simulink model "Campus_Power_System_updated"  (R2024a)
settings: Solver=daessc  StartTime=0.0  StopTime=1  RelTol=1e-3
libraries: spsThreePhaseVIMeasurementLib x57, spsThreePhaseTransformerTwoWindingsLib x56, spsThreePhaseSeriesRLCLoadLib x55, spsThreePhasePISectionLineLib x54, spsThreePhaseBreakerLib x9, spsCurrentMeasurementLib x3, spsMultimeterLib x1, spsThreePhaseSourceLib x1, spsThreePhaseFaultLib x1, sps_lib x1
(part 2 of 3)

== system Campus_Power_System_updated/Engineering (1) ==
  33/11KV Transformer 1 : spsThreePhaseTransformerTwoWindingsLib/Three-Phase Transformer (Two Windings)  Winding1Connection=Yg  Winding2Connection=Yg  CoreType=Three single-phase transformers  SetSaturation=off  Hysteresis=off  DataFile='hysteresis'  SetInitialFlux=off  Measurements=None  UNITS=pu  NominalPower=[ 250e6 , 50 ]  Winding1=[33e3 , 0.002 , 0.08 ]  Winding2=[ 11e3 , 0.002 , 0.08 ]  Rm=500  Lm=500  L0=0.5  Saturation=[ 0,0 ; 0.0024,1.2 ; 1.0,1.52 ]  InitialFluxes=[ 0.8 , -0.8 , 0.7 ]  BreakLoop=off  DiscreteSolver=Trapezoidal iterative  DataType=off  TransfoNumber=1
  BUS1 : spsThreePhaseVIMeasurementLib/Three-Phase V-I Measurement  VoltageMeasurement=phase-to-ground  SetLabelV=off  LabelV=Vabc  Vpu=off  VpuLL=off  CurrentMeasurement=yes  SetLabelI=off  LabelI=Iabc  Ipu=off  Pbase=100e6  Vbase=500e3  OutputType=Complex  PhasorSimulation=off  PSBequivalent=0
  Mux1 : Mux  Inputs=2
  Scope1 : Scope
  Three-Phase Series RLC Load : spsThreePhaseSeriesRLCLoadLib/Three-Phase Series RLC Load  LConnTagsString=A|B|C  Configuration=Y (grounded)  NominalVoltage=1000  Vabc=[1e3 1e3 1e3]  Vabcp=[1e3 1e3 1e3]  NominalFrequency=60  UnbalancedPower=off  ActivePower=10e3  InductivePower=100  CapacitivePower=100  Pabc=[10e3 9e3 11e3]  QLabc=[100 90 110]  QCabc=[100 90 110]  Pabcp=[10e3 9e3 11e3]  QLabcp=[100 90 110]  QCabcp=[100 90 110]  Measurements=None  LoadType=constant Z
  A : PMIOPort  Side=Left
  B : PMIOPort  Port=2  Side=Left
  C : PMIOPort  Port=3  Side=Left
  wires:
  BUS1/2 -> Mux1/2
  BUS1/1 -> Mux1/1
  Mux1/1 -> Scope1/1
  connections:
  33/11KV Transformer 1/RConn3 -- BUS1/LConn3
  33/11KV Transformer 1/RConn1 -- BUS1/LConn1
  BUS1/RConn2 -- Three-Phase Series RLC Load/LConn2
  BUS1/RConn3 -- Three-Phase Series RLC Load/LConn3
  33/11KV Transformer 1/RConn2 -- BUS1/LConn2
  BUS1/RConn1 -- Three-Phase Series RLC Load/LConn1
  33/11KV Transformer 1/LConn1 -- A/RConn1
  33/11KV Transformer 1/LConn3 -- C/RConn1
  33/11KV Transformer 1/LConn2 -- B/RConn1

== system Campus_Power_System_updated/Engineering (ii) ==
  33/11KV Transformer 1 : spsThreePhaseTransformerTwoWindingsLib/Three-Phase Transformer (Two Windings)  Winding1Connection=Yg  Winding2Connection=Yg  CoreType=Three single-phase transformers  SetSaturation=off  Hysteresis=off  DataFile='hysteresis'  SetInitialFlux=off  Measurements=None  UNITS=pu  NominalPower=[ 250e6 , 50 ]  Winding1=[33e3 , 0.002 , 0.08 ]  Winding2=[ 11e3 , 0.002 , 0.08 ]  Rm=500  Lm=500  L0=0.5  Saturation=[ 0,0 ; 0.0024,1.2 ; 1.0,1.52 ]  InitialFluxes=[ 0.8 , -0.8 , 0.7 ]  BreakLoop=off  DiscreteSolver=Trapezoidal iterative  DataType=off  TransfoNumber=1
  BUS1 : spsThreePhaseVIMeasurementLib/Three-Phase V-I Measurement  VoltageMeasurement=phase-to-ground  SetLabelV=off  LabelV=Vabc  Vpu=off  VpuLL=off  CurrentMeasurement=yes  SetLabelI=off  LabelI=Iabc  Ipu=off  Pbase=100e6  Vbase=500e3  OutputType=Complex  PhasorSimulation=off  PSBequivalent=0
  Mux1 : Mux  Inputs=2
  Scope1 : Scope
  Three-Phase Series RLC Load : spsThreePhaseSeriesRLCLoadLib/Three-Phase Series RLC Load  LConnTagsString=A|B|C  Configuration=Y (grounded)  NominalVoltage=1000  Vabc=[1e3 1e3 1e3]  Vabcp=[1e3 1e3 1e3]  NominalFrequency=60  UnbalancedPower=off  ActivePower=10e3  InductivePower=100  CapacitivePower=100  Pabc=[10e3 9e3 11e3]  QLabc=[100 90 110]  QCabc=[100 90 110]  Pabcp=[10e3 9e3 11e3]  QLabcp=[100 90 110]  QCabcp=[100 90 110]  Measurements=None  LoadType=constant Z
  A : PMIOPort  Side=Left
  B : PMIOPort  Port=2  Side=Left
  C : PMIOPort  Port=3  Side=Left
  wires:
  BUS1/2 -> Mux1/2
  BUS1/1 -> Mux1/1
  Mux1/1 -> Scope1/1
  connections:
  33/11KV Transformer 1/RConn3 -- BUS1/LConn3
  33/11KV Transformer 1/RConn1 -- BUS1/LConn1
  BUS1/RConn2 -- Three-Phase Series RLC Load/LConn2
  BUS1/RConn3 -- Three-Phase Series RLC Load/LConn3
  33/11KV Transformer 1/RConn2 -- BUS1/LConn2
  BUS1/RConn1 -- Three-Phase Series RLC Load/LConn1
  33/11KV Transformer 1/LConn1 -- A/RConn1
  33/11KV Transformer 1/LConn3 -- C/RConn1
  33/11KV Transformer 1/LConn2 -- B/RConn1

== system Campus_Power_System_updated/Environmental Science ==
  33/11KV Transformer 1 : spsThreePhaseTransformerTwoWindingsLib/Three-Phase Transformer (Two Windings)  Winding1Connection=Yg  Winding2Connection=Yg  CoreType=Three single-phase transformers  SetSaturation=off  Hysteresis=off  DataFile='hysteresis'  SetInitialFlux=off  Measurements=None  UNITS=pu  NominalPower=[ 250e6 , 50 ]  Winding1=[33e3 , 0.002 , 0.08 ]  Winding2=[ 11e3 , 0.002 , 0.08 ]  Rm=500  Lm=500  L0=0.5  Saturation=[ 0,0 ; 0.0024,1.2 ; 1.0,1.52 ]  InitialFluxes=[ 0.8 , -0.8 , 0.7 ]  BreakLoop=off  DiscreteSolver=Trapezoidal iterative  DataType=off  TransfoNumber=1
  Environmental Science : Scope
  Environmental Science_ : spsThreePhaseVIMeasurementLib/Three-Phase V-I Measurement  VoltageMeasurement=phase-to-ground  SetLabelV=off  LabelV=Vabc  Vpu=off  VpuLL=off  CurrentMeasurement=yes  SetLabelI=off  LabelI=Iabc  Ipu=off  Pbase=100e6  Vbase=500e3  OutputType=Complex  PhasorSimulation=off  PSBequivalent=0
  Mux1 : Mux  Inputs=2
  Three-Phase Series RLC Load : spsThreePhaseSeriesRLCLoadLib/Three-Phase Series RLC Load  LConnTagsString=A|B|C  Configuration=Y (grounded)  NominalVoltage=240  Vabc=[1e3 1e3 1e3]  Vabcp=[1e3 1e3 1e3]  NominalFrequency=50  UnbalancedPower=off  ActivePower=10e3  InductivePower=100  CapacitivePower=100  Pabc=[10e3 9e3 11e3]  QLabc=[100 90 110]  QCabc=[100 90 110]  Pabcp=[10e3 9e3 11e3]  QLabcp=[100 90 110]  QCabcp=[100 90 110]  Measurements=None  LoadType=constant Z
  A : PMIOPort  Side=Left
  B : PMIOPort  Port=2  Side=Left
  C : PMIOPort  Port=3  Side=Left
  wires:
  Environmental Science_/2 -> Mux1/2
  Environmental Science_/1 -> Mux1/1
  Mux1/1 -> Environmental Science/1
  connections:
  33/11KV Transformer 1/RConn3 -- Environmental Science_/LConn3
  33/11KV Transformer 1/RConn1 -- Environmental Science_/LConn1
  Environmental Science_/RConn2 -- Three-Phase Series RLC Load/LConn2
  Environmental Science_/RConn3 -- Three-Phase Series RLC Load/LConn3
  33/11KV Transformer 1/RConn2 -- Environmental Science_/LConn2
  Environmental Science_/RConn1 -- Three-Phase Series RLC Load/LConn1
  33/11KV Transformer 1/LConn1 -- A/RConn1
  33/11KV Transformer 1/LConn3 -- C/RConn1
  33/11KV Transformer 1/LConn2 -- B/RConn1

== system Campus_Power_System_updated/Guest House ==
  33/11KV Transformer 1 : spsThreePhaseTransformerTwoWindingsLib/Three-Phase Transformer (Two Windings)  Winding1Connection=Yg  Winding2Connection=Yg  CoreType=Three single-phase transformers  SetSaturation=off  Hysteresis=off  DataFile='hysteresis'  SetInitialFlux=off  Measurements=None  UNITS=pu  NominalPower=[ 250e6 , 50 ]  Winding1=[33e3 , 0.002 , 0.08 ]  Winding2=[ 11e3 , 0.002 , 0.08 ]  Rm=500  Lm=500  L0=0.5  Saturation=[ 0,0 ; 0.0024,1.2 ; 1.0,1.52 ]  InitialFluxes=[ 0.8 , -0.8 , 0.7 ]  BreakLoop=off  DiscreteSolver=Trapezoidal iterative  DataType=off  TransfoNumber=1
  BUS1 : spsThreePhaseVIMeasurementLib/Three-Phase V-I Measurement  VoltageMeasurement=phase-to-ground  SetLabelV=off  LabelV=Vabc  Vpu=off  VpuLL=off  CurrentMeasurement=yes  SetLabelI=off  LabelI=Iabc  Ipu=off  Pbase=100e6  Vbase=500e3  OutputType=Complex  PhasorSimulation=off  PSBequivalent=0
  Mux1 : Mux  Inputs=2
  Scope1 : Scope
  Three-Phase Series RLC Load : spsThreePhaseSeriesRLCLoadLib/Three-Phase Series RLC Load  LConnTagsString=A|B|C  Configuration=Y (grounded)  NominalVoltage=1000  Vabc=[1e3 1e3 1e3]  Vabcp=[1e3 1e3 1e3]  NominalFrequency=60  UnbalancedPower=off  ActivePower=10e3  InductivePower=100  CapacitivePower=100  Pabc=[10e3 9e3 11e3]  QLabc=[100 90 110]  QCabc=[100 90 110]  Pabcp=[10e3 9e3 11e3]  QLabcp=[100 90 110]  QCabcp=[100 90 110]  Measurements=None  LoadType=constant Z
  A : PMIOPort  Side=Left
  B : PMIOPort  Port=2  Side=Left
  C : PMIOPort  Port=3  Side=Left
  wires:
  BUS1/2 -> Mux1/2
  BUS1/1 -> Mux1/1
  Mux1/1 -> Scope1/1
  connections:
  33/11KV Transformer 1/RConn3 -- BUS1/LConn3
  33/11KV Transformer 1/RConn1 -- BUS1/LConn1
  BUS1/RConn2 -- Three-Phase Series RLC Load/LConn2
  BUS1/RConn3 -- Three-Phase Series RLC Load/LConn3
  33/11KV Transformer 1/RConn2 -- BUS1/LConn2
  BUS1/RConn1 -- Three-Phase Series RLC Load/LConn1
  33/11KV Transformer 1/LConn1 -- A/RConn1
  33/11KV Transformer 1/LConn3 -- C/RConn1
  33/11KV Transformer 1/LConn2 -- B/RConn1

== system Campus_Power_System_updated/HRDB ==
  33/11KV Transformer 1 : spsThreePhaseTransformerTwoWindingsLib/Three-Phase Transformer (Two Windings)  Winding1Connection=Yg  Winding2Connection=Yg  CoreType=Three single-phase transformers  SetSaturation=off  Hysteresis=off  DataFile='hysteresis'  SetInitialFlux=off  Measurements=None  UNITS=pu  NominalPower=[ 250e6 , 50 ]  Winding1=[33e3 , 0.002 , 0.08 ]  Winding2=[ 11e3 , 0.002 , 0.08 ]  Rm=500  Lm=500  L0=0.5  Saturation=[ 0,0 ; 0.0024,1.2 ; 1.0,1.52 ]  InitialFluxes=[ 0.8 , -0.8 , 0.7 ]  BreakLoop=off  DiscreteSolver=Trapezoidal iterative  DataType=off  TransfoNumber=1
  BUS1 : spsThreePhaseVIMeasurementLib/Three-Phase V-I Measurement  VoltageMeasurement=phase-to-ground  SetLabelV=off  LabelV=Vabc  Vpu=off  VpuLL=off  CurrentMeasurement=yes  SetLabelI=off  LabelI=Iabc  Ipu=off  Pbase=100e6  Vbase=500e3  OutputType=Complex  PhasorSimulation=off  PSBequivalent=0
  Mux1 : Mux  Inputs=2
  Scope1 : Scope
  Three-Phase Series RLC Load : spsThreePhaseSeriesRLCLoadLib/Three-Phase Series RLC Load  LConnTagsString=A|B|C  Configuration=Y (grounded)  NominalVoltage=1000  Vabc=[1e3 1e3 1e3]  Vabcp=[1e3 1e3 1e3]  NominalFrequency=60  UnbalancedPower=off  ActivePower=10e3  InductivePower=100  CapacitivePower=100  Pabc=[10e3 9e3 11e3]  QLabc=[100 90 110]  QCabc=[100 90 110]  Pabcp=[10e3 9e3 11e3]  QLabcp=[100 90 110]  QCabcp=[100 90 110]  Measurements=None  LoadType=constant Z
  A : PMIOPort  Side=Left
  B : PMIOPort  Port=2  Side=Left
  C : PMIOPort  Port=3  Side=Left
  wires:
  BUS1/2 -> Mux1/2
  BUS1/1 -> Mux1/1
  Mux1/1 -> Scope1/1
  connections:
  33/11KV Transformer 1/RConn3 -- BUS1/LConn3
  33/11KV Transformer 1/RConn1 -- BUS1/LConn1
  BUS1/RConn2 -- Three-Phase Series RLC Load/LConn2
  BUS1/RConn3 -- Three-Phase Series RLC Load/LConn3
  33/11KV Transformer 1/RConn2 -- BUS1/LConn2
  BUS1/RConn1 -- Three-Phase Series RLC Load/LConn1
  33/11KV Transformer 1/LConn1 -- A/RConn1
  33/11KV Transformer 1/LConn3 -- C/RConn1
  33/11KV Transformer 1/LConn2 -- B/RConn1

== system Campus_Power_System_updated/HV laboratory ==
  33/11KV Transformer 1 : spsThreePhaseTransformerTwoWindingsLib/Three-Phase Transformer (Two Windings)  Winding1Connection=Yg  Winding2Connection=Yg  CoreType=Three single-phase transformers  SetSaturation=off  Hysteresis=off  DataFile='hysteresis'  SetInitialFlux=off  Measurements=None  UNITS=pu  NominalPower=[ 250e6 , 50 ]  Winding1=[33e3 , 0.002 , 0.08 ]  Winding2=[ 11e3 , 0.002 , 0.08 ]  Rm=500  Lm=500  L0=0.5  Saturation=[ 0,0 ; 0.0024,1.2 ; 1.0,1.52 ]  InitialFluxes=[ 0.8 , -0.8 , 0.7 ]  BreakLoop=off  DiscreteSolver=Trapezoidal iterative  DataType=off  TransfoNumber=1
  BUS1 : spsThreePhaseVIMeasurementLib/Three-Phase V-I Measurement  VoltageMeasurement=phase-to-ground  SetLabelV=off  LabelV=Vabc  Vpu=off  VpuLL=off  CurrentMeasurement=yes  SetLabelI=off  LabelI=Iabc  Ipu=off  Pbase=100e6  Vbase=500e3  OutputType=Complex  PhasorSimulation=off  PSBequivalent=0
  Mux1 : Mux  Inputs=2
  Scope1 : Scope
  Three-Phase Series RLC Load : spsThreePhaseSeriesRLCLoadLib/Three-Phase Series RLC Load  LConnTagsString=A|B|C  Configuration=Y (grounded)  NominalVoltage=1000  Vabc=[1e3 1e3 1e3]  Vabcp=[1e3 1e3 1e3]  NominalFrequency=60  UnbalancedPower=off  ActivePower=10e3  InductivePower=100  CapacitivePower=100  Pabc=[10e3 9e3 11e3]  QLabc=[100 90 110]  QCabc=[100 90 110]  Pabcp=[10e3 9e3 11e3]  QLabcp=[100 90 110]  QCabcp=[100 90 110]  Measurements=None  LoadType=constant Z
  A : PMIOPort  Side=Left
  B : PMIOPort  Port=2  Side=Left
  C : PMIOPort  Port=3  Side=Left
  wires:
  BUS1/2 -> Mux1/2
  BUS1/1 -> Mux1/1
  Mux1/1 -> Scope1/1
  connections:
  33/11KV Transformer 1/RConn3 -- BUS1/LConn3
  33/11KV Transformer 1/RConn1 -- BUS1/LConn1
  BUS1/RConn2 -- Three-Phase Series RLC Load/LConn2
  BUS1/RConn3 -- Three-Phase Series RLC Load/LConn3
  33/11KV Transformer 1/RConn2 -- BUS1/LConn2
  BUS1/RConn1 -- Three-Phase Series RLC Load/LConn1
  33/11KV Transformer 1/LConn1 -- A/RConn1
  33/11KV Transformer 1/LConn3 -- C/RConn1
  33/11KV Transformer 1/LConn2 -- B/RConn1

== system Campus_Power_System_updated/Health Centre ==
  33/11KV Transformer 1 : spsThreePhaseTransformerTwoWindingsLib/Three-Phase Transformer (Two Windings)  Winding1Connection=Yg  Winding2Connection=Yg  CoreType=Three single-phase transformers  SetSaturation=off  Hysteresis=off  DataFile='hysteresis'  SetInitialFlux=off  Measurements=None  UNITS=pu  NominalPower=[ 250e6 , 50 ]  Winding1=[33e3 , 0.002 , 0.08 ]  Winding2=[ 11e3 , 0.002 , 0.08 ]  Rm=500  Lm=500  L0=0.5  Saturation=[ 0,0 ; 0.0024,1.2 ; 1.0,1.52 ]  InitialFluxes=[ 0.8 , -0.8 , 0.7 ]  BreakLoop=off  DiscreteSolver=Trapezoidal iterative  DataType=off  TransfoNumber=1
  BUS1 : spsThreePhaseVIMeasurementLib/Three-Phase V-I Measurement  VoltageMeasurement=phase-to-ground  SetLabelV=off  LabelV=Vabc  Vpu=off  VpuLL=off  CurrentMeasurement=yes  SetLabelI=off  LabelI=Iabc  Ipu=off  Pbase=100e6  Vbase=500e3  OutputType=Complex  PhasorSimulation=off  PSBequivalent=0
  Mux1 : Mux  Inputs=2
  Scope1 : Scope
  Three-Phase Series RLC Load : spsThreePhaseSeriesRLCLoadLib/Three-Phase Series RLC Load  LConnTagsString=A|B|C  Configuration=Y (grounded)  NominalVoltage=1000  Vabc=[1e3 1e3 1e3]  Vabcp=[1e3 1e3 1e3]  NominalFrequency=60  UnbalancedPower=off  ActivePower=10e3  InductivePower=100  CapacitivePower=100  Pabc=[10e3 9e3 11e3]  QLabc=[100 90 110]  QCabc=[100 90 110]  Pabcp=[10e3 9e3 11e3]  QLabcp=[100 90 110]  QCabcp=[100 90 110]  Measurements=None  LoadType=constant Z
  A : PMIOPort  Side=Left
  B : PMIOPort  Port=2  Side=Left
  C : PMIOPort  Port=3  Side=Left
  wires:
  BUS1/2 -> Mux1/2
  BUS1/1 -> Mux1/1
  Mux1/1 -> Scope1/1
  connections:
  33/11KV Transformer 1/RConn3 -- BUS1/LConn3
  33/11KV Transformer 1/RConn1 -- BUS1/LConn1
  BUS1/RConn2 -- Three-Phase Series RLC Load/LConn2
  BUS1/RConn3 -- Three-Phase Series RLC Load/LConn3
  33/11KV Transformer 1/RConn2 -- BUS1/LConn2
  BUS1/RConn1 -- Three-Phase Series RLC Load/LConn1
  33/11KV Transformer 1/LConn1 -- A/RConn1
  33/11KV Transformer 1/LConn3 -- C/RConn1
  33/11KV Transformer 1/LConn2 -- B/RConn1

== system Campus_Power_System_updated/Henry cafe ==
  33/11KV Transformer 1 : spsThreePhaseTransformerTwoWindingsLib/Three-Phase Transformer (Two Windings)  Winding1Connection=Yg  Winding2Connection=Yg  CoreType=Three single-phase transformers  SetSaturation=off  Hysteresis=off  DataFile='hysteresis'  SetInitialFlux=off  Measurements=None  UNITS=pu  NominalPower=[ 250e6 , 50 ]  Winding1=[33e3 , 0.002 , 0.08 ]  Winding2=[ 11e3 , 0.002 , 0.08 ]  Rm=500  Lm=500  L0=0.5  Saturation=[ 0,0 ; 0.0024,1.2 ; 1.0,1.52 ]  InitialFluxes=[ 0.8 , -0.8 , 0.7 ]  BreakLoop=off  DiscreteSolver=Trapezoidal iterative  DataType=off  TransfoNumber=1
  BUS1 : spsThreePhaseVIMeasurementLib/Three-Phase V-I Measurement  VoltageMeasurement=phase-to-ground  SetLabelV=off  LabelV=Vabc  Vpu=off  VpuLL=off  CurrentMeasurement=yes  SetLabelI=off  LabelI=Iabc  Ipu=off  Pbase=100e6  Vbase=500e3  OutputType=Complex  PhasorSimulation=off  PSBequivalent=0
  Mux1 : Mux  Inputs=2
  Scope1 : Scope
  Three-Phase Series RLC Load : spsThreePhaseSeriesRLCLoadLib/Three-Phase Series RLC Load  LConnTagsString=A|B|C  Configuration=Y (grounded)  NominalVoltage=1000  Vabc=[1e3 1e3 1e3]  Vabcp=[1e3 1e3 1e3]  NominalFrequency=60  UnbalancedPower=off  ActivePower=10e3  InductivePower=100  CapacitivePower=100  Pabc=[10e3 9e3 11e3]  QLabc=[100 90 110]  QCabc=[100 90 110]  Pabcp=[10e3 9e3 11e3]  QLabcp=[100 90 110]  QCabcp=[100 90 110]  Measurements=None  LoadType=constant Z
  A : PMIOPort  Side=Left
  B : PMIOPort  Port=2  Side=Left
  C : PMIOPort  Port=3  Side=Left
  wires:
  BUS1/2 -> Mux1/2
  BUS1/1 -> Mux1/1
  Mux1/1 -> Scope1/1
  connections:
  33/11KV Transformer 1/RConn3 -- BUS1/LConn3
  33/11KV Transformer 1/RConn1 -- BUS1/LConn1
  BUS1/RConn2 -- Three-Phase Series RLC Load/LConn2
  BUS1/RConn3 -- Three-Phase Series RLC Load/LConn3
  33/11KV Transformer 1/RConn2 -- BUS1/LConn2
  BUS1/RConn1 -- Three-Phase Series RLC Load/LConn1
  33/11KV Transformer 1/LConn1 -- A/RConn1
  33/11KV Transformer 1/LConn3 -- C/RConn1
  33/11KV Transformer 1/LConn2 -- B/RConn1

== system Campus_Power_System_updated/High Rise Block (Auxilliary) ==
  33/11KV Transformer 1 : spsThreePhaseTransformerTwoWindingsLib/Three-Phase Transformer (Two Windings)  Winding1Connection=Yg  Winding2Connection=Yg  CoreType=Three single-phase transformers  SetSaturation=off  Hysteresis=off  DataFile='hysteresis'  SetInitialFlux=off  Measurements=None  UNITS=pu  NominalPower=[ 250e6 , 50 ]  Winding1=[33e3 , 0.002 , 0.08 ]  Winding2=[ 11e3 , 0.002 , 0.08 ]  Rm=500  Lm=500  L0=0.5  Saturation=[ 0,0 ; 0.0024,1.2 ; 1.0,1.52 ]  InitialFluxes=[ 0.8 , -0.8 , 0.7 ]  BreakLoop=off  DiscreteSolver=Trapezoidal iterative  DataType=off  TransfoNumber=1
  BUS1 : spsThreePhaseVIMeasurementLib/Three-Phase V-I Measurement  VoltageMeasurement=phase-to-ground  SetLabelV=off  LabelV=Vabc  Vpu=off  VpuLL=off  CurrentMeasurement=yes  SetLabelI=off  LabelI=Iabc  Ipu=off  Pbase=100e6  Vbase=500e3  OutputType=Complex  PhasorSimulation=off  PSBequivalent=0
  Mux1 : Mux  Inputs=2
  Scope1 : Scope
  Three-Phase Series RLC Load : spsThreePhaseSeriesRLCLoadLib/Three-Phase Series RLC Load  LConnTagsString=A|B|C  Configuration=Y (grounded)  NominalVoltage=1000  Vabc=[1e3 1e3 1e3]  Vabcp=[1e3 1e3 1e3]  NominalFrequency=60  UnbalancedPower=off  ActivePower=10e3  InductivePower=100  CapacitivePower=100  Pabc=[10e3 9e3 11e3]  QLabc=[100 90 110]  QCabc=[100 90 110]  Pabcp=[10e3 9e3 11e3]  QLabcp=[100 90 110]  QCabcp=[100 90 110]  Measurements=None  LoadType=constant Z
  A : PMIOPort  Side=Left
  B : PMIOPort  Port=2  Side=Left
  C : PMIOPort  Port=3  Side=Left
  wires:
  BUS1/2 -> Mux1/2
  BUS1/1 -> Mux1/1
  Mux1/1 -> Scope1/1
  connections:
  33/11KV Transformer 1/RConn3 -- BUS1/LConn3
  33/11KV Transformer 1/RConn1 -- BUS1/LConn1
  BUS1/RConn2 -- Three-Phase Series RLC Load/LConn2
  BUS1/RConn3 -- Three-Phase Series RLC Load/LConn3
  33/11KV Transformer 1/RConn2 -- BUS1/LConn2
  BUS1/RConn1 -- Three-Phase Series RLC Load/LConn1
  33/11KV Transformer 1/LConn1 -- A/RConn1
  33/11KV Transformer 1/LConn3 -- C/RConn1
  33/11KV Transformer 1/LConn2 -- B/RConn1

== system Campus_Power_System_updated/High Rise Block A ==
  33/11KV Transformer 1 : spsThreePhaseTransformerTwoWindingsLib/Three-Phase Transformer (Two Windings)  Winding1Connection=Yg  Winding2Connection=Yg  CoreType=Three single-phase transformers  SetSaturation=off  Hysteresis=off  DataFile='hysteresis'  SetInitialFlux=off  Measurements=None  UNITS=pu  NominalPower=[ 250e6 , 50 ]  Winding1=[33e3 , 0.002 , 0.08 ]  Winding2=[ 11e3 , 0.002 , 0.08 ]  Rm=500  Lm=500  L0=0.5  Saturation=[ 0,0 ; 0.0024,1.2 ; 1.0,1.52 ]  InitialFluxes=[ 0.8 , -0.8 , 0.7 ]  BreakLoop=off  DiscreteSolver=Trapezoidal iterative  DataType=off  TransfoNumber=1
  BUS1 : spsThreePhaseVIMeasurementLib/Three-Phase V-I Measurement  VoltageMeasurement=phase-to-ground  SetLabelV=off  LabelV=Vabc  Vpu=off  VpuLL=off  CurrentMeasurement=yes  SetLabelI=off  LabelI=Iabc  Ipu=off  Pbase=100e6  Vbase=500e3  OutputType=Complex  PhasorSimulation=off  PSBequivalent=0
  Mux1 : Mux  Inputs=2
  Scope1 : Scope
  Three-Phase Series RLC Load : spsThreePhaseSeriesRLCLoadLib/Three-Phase Series RLC Load  LConnTagsString=A|B|C  Configuration=Y (grounded)  NominalVoltage=1000  Vabc=[1e3 1e3 1e3]  Vabcp=[1e3 1e3 1e3]  NominalFrequency=60  UnbalancedPower=off  ActivePower=10e3  InductivePower=100  CapacitivePower=100  Pabc=[10e3 9e3 11e3]  QLabc=[100 90 110]  QCabc=[100 90 110]  Pabcp=[10e3 9e3 11e3]  QLabcp=[100 90 110]  QCabcp=[100 90 110]  Measurements=None  LoadType=constant Z
  A : PMIOPort  Side=Left
  B : PMIOPort  Port=2  Side=Left
  C : PMIOPort  Port=3  Side=Left
  wires:
  BUS1/2 -> Mux1/2
  BUS1/1 -> Mux1/1
  Mux1/1 -> Scope1/1
  connections:
  33/11KV Transformer 1/RConn3 -- BUS1/LConn3
  33/11KV Transformer 1/RConn1 -- BUS1/LConn1
  BUS1/RConn2 -- Three-Phase Series RLC Load/LConn2
  BUS1/RConn3 -- Three-Phase Series RLC Load/LConn3
  33/11KV Transformer 1/RConn2 -- BUS1/LConn2
  BUS1/RConn1 -- Three-Phase Series RLC Load/LConn1
  33/11KV Transformer 1/LConn1 -- A/RConn1
  33/11KV Transformer 1/LConn3 -- C/RConn1
  33/11KV Transformer 1/LConn2 -- B/RConn1

== system Campus_Power_System_updated/High Rise Block B ==
  33/11KV Transformer 1 : spsThreePhaseTransformerTwoWindingsLib/Three-Phase Transformer (Two Windings)  Winding1Connection=Yg  Winding2Connection=Yg  CoreType=Three single-phase transformers  SetSaturation=off  Hysteresis=off  DataFile='hysteresis'  SetInitialFlux=off  Measurements=None  UNITS=pu  NominalPower=[ 250e6 , 50 ]  Winding1=[33e3 , 0.002 , 0.08 ]  Winding2=[ 11e3 , 0.002 , 0.08 ]  Rm=500  Lm=500  L0=0.5  Saturation=[ 0,0 ; 0.0024,1.2 ; 1.0,1.52 ]  InitialFluxes=[ 0.8 , -0.8 , 0.7 ]  BreakLoop=off  DiscreteSolver=Trapezoidal iterative  DataType=off  TransfoNumber=1
  BUS1 : spsThreePhaseVIMeasurementLib/Three-Phase V-I Measurement  VoltageMeasurement=phase-to-ground  SetLabelV=off  LabelV=Vabc  Vpu=off  VpuLL=off  CurrentMeasurement=yes  SetLabelI=off  LabelI=Iabc  Ipu=off  Pbase=100e6  Vbase=500e3  OutputType=Complex  PhasorSimulation=off  PSBequivalent=0
  Mux1 : Mux  Inputs=2
  Scope1 : Scope
  Three-Phase Series RLC Load : spsThreePhaseSeriesRLCLoadLib/Three-Phase Series RLC Load  LConnTagsString=A|B|C  Configuration=Y (grounded)  NominalVoltage=1000  Vabc=[1e3 1e3 1e3]  Vabcp=[1e3 1e3 1e3]  NominalFrequency=60  UnbalancedPower=off  ActivePower=10e3  InductivePower=100  CapacitivePower=100  Pabc=[10e3 9e3 11e3]  QLabc=[100 90 110]  QCabc=[100 90 110]  Pabcp=[10e3 9e3 11e3]  QLabcp=[100 90 110]  QCabcp=[100 90 110]  Measurements=None  LoadType=constant Z
  A : PMIOPort  Side=Left
  B : PMIOPort  Port=2  Side=Left
  C : PMIOPort  Port=3  Side=Left
  wires:
  BUS1/2 -> Mux1/2
  BUS1/1 -> Mux1/1
  Mux1/1 -> Scope1/1
  connections:
  33/11KV Transformer 1/RConn3 -- BUS1/LConn3
  33/11KV Transformer 1/RConn1 -- BUS1/LConn1
  BUS1/RConn2 -- Three-Phase Series RLC Load/LConn2
  BUS1/RConn3 -- Three-Phase Series RLC Load/LConn3
  33/11KV Transformer 1/RConn2 -- BUS1/LConn2
  BUS1/RConn1 -- Three-Phase Series RLC Load/LConn1
  33/11KV Transformer 1/LConn1 -- A/RConn1
  33/11KV Transformer 1/LConn3 -- C/RConn1
  33/11KV Transformer 1/LConn2 -- B/RConn1

== system Campus_Power_System_updated/High Rise Block C ==
  33/11KV Transformer 1 : spsThreePhaseTransformerTwoWindingsLib/Three-Phase Transformer (Two Windings)  Winding1Connection=Yg  Winding2Connection=Yg  CoreType=Three single-phase transformers  SetSaturation=off  Hysteresis=off  DataFile='hysteresis'  SetInitialFlux=off  Measurements=None  UNITS=pu  NominalPower=[ 250e6 , 50 ]  Winding1=[33e3 , 0.002 , 0.08 ]  Winding2=[ 11e3 , 0.002 , 0.08 ]  Rm=500  Lm=500  L0=0.5  Saturation=[ 0,0 ; 0.0024,1.2 ; 1.0,1.52 ]  InitialFluxes=[ 0.8 , -0.8 , 0.7 ]  BreakLoop=off  DiscreteSolver=Trapezoidal iterative  DataType=off  TransfoNumber=1
  BUS1 : spsThreePhaseVIMeasurementLib/Three-Phase V-I Measurement  VoltageMeasurement=phase-to-ground  SetLabelV=off  LabelV=Vabc  Vpu=off  VpuLL=off  CurrentMeasurement=yes  SetLabelI=off  LabelI=Iabc  Ipu=off  Pbase=100e6  Vbase=500e3  OutputType=Complex  PhasorSimulation=off  PSBequivalent=0
  Mux1 : Mux  Inputs=2
  Scope1 : Scope
  Three-Phase Series RLC Load : spsThreePhaseSeriesRLCLoadLib/Three-Phase Series RLC Load  LConnTagsString=A|B|C  Configuration=Y (grounded)  NominalVoltage=1000  Vabc=[1e3 1e3 1e3]  Vabcp=[1e3 1e3 1e3]  NominalFrequency=60  UnbalancedPower=off  ActivePower=10e3  InductivePower=100  CapacitivePower=100  Pabc=[10e3 9e3 11e3]  QLabc=[100 90 110]  QCabc=[100 90 110]  Pabcp=[10e3 9e3 11e3]  QLabcp=[100 90 110]  QCabcp=[100 90 110]  Measurements=None  LoadType=constant Z
  A : PMIOPort  Side=Left
  B : PMIOPort  Port=2  Side=Left
  C : PMIOPort  Port=3  Side=Left
  wires:
  BUS1/2 -> Mux1/2
  BUS1/1 -> Mux1/1
  Mux1/1 -> Scope1/1
  connections:
  33/11KV Transformer 1/RConn3 -- BUS1/LConn3
  33/11KV Transformer 1/RConn1 -- BUS1/LConn1
  BUS1/RConn2 -- Three-Phase Series RLC Load/LConn2
  BUS1/RConn3 -- Three-Phase Series RLC Load/LConn3
  33/11KV Transformer 1/RConn2 -- BUS1/LConn2
  BUS1/RConn1 -- Three-Phase Series RLC Load/LConn1
  33/11KV Transformer 1/LConn1 -- A/RConn1
  33/11KV Transformer 1/LConn3 -- C/RConn1
  33/11KV Transformer 1/LConn2 -- B/RConn1

== system Campus_Power_System_updated/Hydraulic Research Centre ==
  33/11KV Transformer 1 : spsThreePhaseTransformerTwoWindingsLib/Three-Phase Transformer (Two Windings)  Winding1Connection=Yg  Winding2Connection=Yg  CoreType=Three single-phase transformers  SetSaturation=off  Hysteresis=off  DataFile='hysteresis'  SetInitialFlux=off  Measurements=None  UNITS=pu  NominalPower=[ 250e6 , 50 ]  Winding1=[33e3 , 0.002 , 0.08 ]  Winding2=[ 11e3 , 0.002 , 0.08 ]  Rm=500  Lm=500  L0=0.5  Saturation=[ 0,0 ; 0.0024,1.2 ; 1.0,1.52 ]  InitialFluxes=[ 0.8 , -0.8 , 0.7 ]  BreakLoop=off  DiscreteSolver=Trapezoidal iterative  DataType=off  TransfoNumber=1
  BUS1 : spsThreePhaseVIMeasurementLib/Three-Phase V-I Measurement  VoltageMeasurement=phase-to-ground  SetLabelV=off  LabelV=Vabc  Vpu=off  VpuLL=off  CurrentMeasurement=yes  SetLabelI=off  LabelI=Iabc  Ipu=off  Pbase=100e6  Vbase=500e3  OutputType=Complex  PhasorSimulation=off  PSBequivalent=0
  Mux1 : Mux  Inputs=2
  Scope1 : Scope
  Three-Phase Series RLC Load : spsThreePhaseSeriesRLCLoadLib/Three-Phase Series RLC Load  LConnTagsString=A|B|C  Configuration=Y (grounded)  NominalVoltage=1000  Vabc=[1e3 1e3 1e3]  Vabcp=[1e3 1e3 1e3]  NominalFrequency=60  UnbalancedPower=off  ActivePower=10e3  InductivePower=100  CapacitivePower=100  Pabc=[10e3 9e3 11e3]  QLabc=[100 90 110]  QCabc=[100 90 110]  Pabcp=[10e3 9e3 11e3]  QLabcp=[100 90 110]  QCabcp=[100 90 110]  Measurements=None  LoadType=constant Z
  A : PMIOPort  Side=Left
  B : PMIOPort  Port=2  Side=Left
  C : PMIOPort  Port=3  Side=Left
  wires:
  BUS1/2 -> Mux1/2
  BUS1/1 -> Mux1/1
  Mux1/1 -> Scope1/1
  connections:
  33/11KV Transformer 1/RConn3 -- BUS1/LConn3
  33/11KV Transformer 1/RConn1 -- BUS1/LConn1
  BUS1/RConn2 -- Three-Phase Series RLC Load/LConn2
  BUS1/RConn3 -- Three-Phase Series RLC Load/LConn3
  33/11KV Transformer 1/RConn2 -- BUS1/LConn2
  BUS1/RConn1 -- Three-Phase Series RLC Load/LConn1
  33/11KV Transformer 1/LConn1 -- A/RConn1
  33/11KV Transformer 1/LConn3 -- C/RConn1
  33/11KV Transformer 1/LConn2 -- B/RConn1

== system Campus_Power_System_updated/Intercontinental Bank ==
  33/11KV Transformer 1 : spsThreePhaseTransformerTwoWindingsLib/Three-Phase Transformer (Two Windings)  Winding1Connection=Yg  Winding2Connection=Yg  CoreType=Three single-phase transformers  SetSaturation=off  Hysteresis=off  DataFile='hysteresis'  SetInitialFlux=off  Measurements=None  UNITS=pu  NominalPower=[ 250e6 , 50 ]  Winding1=[33e3 , 0.002 , 0.08 ]  Winding2=[ 11e3 , 0.002 , 0.08 ]  Rm=500  Lm=500  L0=0.5  Saturation=[ 0,0 ; 0.0024,1.2 ; 1.0,1.52 ]  InitialFluxes=[ 0.8 , -0.8 , 0.7 ]  BreakLoop=off  DiscreteSolver=Trapezoidal iterative  DataType=off  TransfoNumber=1
  BUS1 : spsThreePhaseVIMeasurementLib/Three-Phase V-I Measurement  VoltageMeasurement=phase-to-ground  SetLabelV=off  LabelV=Vabc  Vpu=off  VpuLL=off  CurrentMeasurement=yes  SetLabelI=off  LabelI=Iabc  Ipu=off  Pbase=100e6  Vbase=500e3  OutputType=Complex  PhasorSimulation=off  PSBequivalent=0
  Mux1 : Mux  Inputs=2
  Scope1 : Scope
  Three-Phase Series RLC Load : spsThreePhaseSeriesRLCLoadLib/Three-Phase Series RLC Load  LConnTagsString=A|B|C  Configuration=Y (grounded)  NominalVoltage=1000  Vabc=[1e3 1e3 1e3]  Vabcp=[1e3 1e3 1e3]  NominalFrequency=60  UnbalancedPower=off  ActivePower=10e3  InductivePower=100  CapacitivePower=100  Pabc=[10e3 9e3 11e3]  QLabc=[100 90 110]  QCabc=[100 90 110]  Pabcp=[10e3 9e3 11e3]  QLabcp=[100 90 110]  QCabcp=[100 90 110]  Measurements=None  LoadType=constant Z
  A : PMIOPort  Side=Left
  B : PMIOPort  Port=2  Side=Left
  C : PMIOPort  Port=3  Side=Left
  wires:
  BUS1/2 -> Mux1/2
  BUS1/1 -> Mux1/1
  Mux1/1 -> Scope1/1
  connections:
  33/11KV Transformer 1/RConn3 -- BUS1/LConn3
  33/11KV Transformer 1/RConn1 -- BUS1/LConn1
  BUS1/RConn2 -- Three-Phase Series RLC Load/LConn2
  BUS1/RConn3 -- Three-Phase Series RLC Load/LConn3
  33/11KV Transformer 1/RConn2 -- BUS1/LConn2
  BUS1/RConn1 -- Three-Phase Series RLC Load/LConn1
  33/11KV Transformer 1/LConn1 -- A/RConn1
  33/11KV Transformer 1/LConn3 -- C/RConn1
  33/11KV Transformer 1/LConn2 -- B/RConn1

== system Campus_Power_System_updated/International School ==
  33/11KV Transformer 1 : spsThreePhaseTransformerTwoWindingsLib/Three-Phase Transformer (Two Windings)  Winding1Connection=Yg  Winding2Connection=Yg  CoreType=Three single-phase transformers  SetSaturation=off  Hysteresis=off  DataFile='hysteresis'  SetInitialFlux=off  Measurements=None  UNITS=pu  NominalPower=[ 250e6 , 50 ]  Winding1=[33e3 , 0.002 , 0.08 ]  Winding2=[ 11e3 , 0.002 , 0.08 ]  Rm=500  Lm=500  L0=0.5  Saturation=[ 0,0 ; 0.0024,1.2 ; 1.0,1.52 ]  InitialFluxes=[ 0.8 , -0.8 , 0.7 ]  BreakLoop=off  DiscreteSolver=Trapezoidal iterative  DataType=off  TransfoNumber=1
  BUS1 : spsThreePhaseVIMeasurementLib/Three-Phase V-I Measurement  VoltageMeasurement=phase-to-ground  SetLabelV=off  LabelV=Vabc  Vpu=off  VpuLL=off  CurrentMeasurement=yes  SetLabelI=off  LabelI=Iabc  Ipu=off  Pbase=100e6  Vbase=500e3  OutputType=Complex  PhasorSimulation=off  PSBequivalent=0
  Mux1 : Mux  Inputs=2
  Scope1 : Scope
  Three-Phase Series RLC Load : spsThreePhaseSeriesRLCLoadLib/Three-Phase Series RLC Load  LConnTagsString=A|B|C  Configuration=Y (grounded)  NominalVoltage=1000  Vabc=[1e3 1e3 1e3]  Vabcp=[1e3 1e3 1e3]  NominalFrequency=60  UnbalancedPower=off  ActivePower=10e3  InductivePower=100  CapacitivePower=100  Pabc=[10e3 9e3 11e3]  QLabc=[100 90 110]  QCabc=[100 90 110]  Pabcp=[10e3 9e3 11e3]  QLabcp=[100 90 110]  QCabcp=[100 90 110]  Measurements=None  LoadType=constant Z
  A : PMIOPort  Side=Left
  B : PMIOPort  Port=2  Side=Left
  C : PMIOPort  Port=3  Side=Left
  wires:
  BUS1/2 -> Mux1/2
  BUS1/1 -> Mux1/1
  Mux1/1 -> Scope1/1
  connections:
  33/11KV Transformer 1/RConn3 -- BUS1/LConn3
  33/11KV Transformer 1/RConn1 -- BUS1/LConn1
  BUS1/RConn2 -- Three-Phase Series RLC Load/LConn2
  BUS1/RConn3 -- Three-Phase Series RLC Load/LConn3
  33/11KV Transformer 1/RConn2 -- BUS1/LConn2
  BUS1/RConn1 -- Three-Phase Series RLC Load/LConn1
  33/11KV Transformer 1/LConn1 -- A/RConn1
  33/11KV Transformer 1/LConn3 -- C/RConn1
  33/11KV Transformer 1/LConn2 -- B/RConn1

== system Campus_Power_System_updated/Jaja Hall ==
  33/11KV Transformer 1 : spsThreePhaseTransformerTwoWindingsLib/Three-Phase Transformer (Two Windings)  Winding1Connection=Yg  Winding2Connection=Yg  CoreType=Three single-phase transformers  SetSaturation=off  Hysteresis=off  DataFile='hysteresis'  SetInitialFlux=off  Measurements=None  UNITS=pu  NominalPower=[ 250e6 , 50 ]  Winding1=[33e3 , 0.002 , 0.08 ]  Winding2=[ 11e3 , 0.002 , 0.08 ]  Rm=500  Lm=500  L0=0.5  Saturation=[ 0,0 ; 0.0024,1.2 ; 1.0,1.52 ]  InitialFluxes=[ 0.8 , -0.8 , 0.7 ]  BreakLoop=off  DiscreteSolver=Trapezoidal iterative  DataType=off  TransfoNumber=1
  BUS1 : spsThreePhaseVIMeasurementLib/Three-Phase V-I Measurement  VoltageMeasurement=phase-to-ground  SetLabelV=off  LabelV=Vabc  Vpu=off  VpuLL=off  CurrentMeasurement=yes  SetLabelI=off  LabelI=Iabc  Ipu=off  Pbase=100e6  Vbase=500e3  OutputType=Complex  PhasorSimulation=off  PSBequivalent=0
  Mux1 : Mux  Inputs=2
  Scope1 : Scope
  Three-Phase Series RLC Load : spsThreePhaseSeriesRLCLoadLib/Three-Phase Series RLC Load  LConnTagsString=A|B|C  Configuration=Y (grounded)  NominalVoltage=1000  Vabc=[1e3 1e3 1e3]  Vabcp=[1e3 1e3 1e3]  NominalFrequency=60  UnbalancedPower=off  ActivePower=10e3  InductivePower=100  CapacitivePower=100  Pabc=[10e3 9e3 11e3]  QLabc=[100 90 110]  QCabc=[100 90 110]  Pabcp=[10e3 9e3 11e3]  QLabcp=[100 90 110]  QCabcp=[100 90 110]  Measurements=None  LoadType=constant Z
  A : PMIOPort  Side=Left
  B : PMIOPort  Port=2  Side=Left
  C : PMIOPort  Port=3  Side=Left
  wires:
  BUS1/2 -> Mux1/2
  BUS1/1 -> Mux1/1
  Mux1/1 -> Scope1/1
  connections:
  33/11KV Transformer 1/RConn3 -- BUS1/LConn3
  33/11KV Transformer 1/RConn1 -- BUS1/LConn1
  BUS1/RConn2 -- Three-Phase Series RLC Load/LConn2
  BUS1/RConn3 -- Three-Phase Series RLC Load/LConn3
  33/11KV Transformer 1/RConn2 -- BUS1/LConn2
  BUS1/RConn1 -- Three-Phase Series RLC Load/LConn1
  33/11KV Transformer 1/LConn1 -- A/RConn1
  33/11KV Transformer 1/LConn3 -- C/RConn1
  33/11KV Transformer 1/LConn2 -- B/RConn1

== system Campus_Power_System_updated/Kosoko Drive ==
  33/11KV Transformer 1 : spsThreePhaseTransformerTwoWindingsLib/Three-Phase Transformer (Two Windings)  Winding1Connection=Yg  Winding2Connection=Yg  CoreType=Three single-phase transformers  SetSaturation=off  Hysteresis=off  DataFile='hysteresis'  SetInitialFlux=off  Measurements=None  UNITS=pu  NominalPower=[ 250e6 , 50 ]  Winding1=[33e3 , 0.002 , 0.08 ]  Winding2=[ 11e3 , 0.002 , 0.08 ]  Rm=500  Lm=500  L0=0.5  Saturation=[ 0,0 ; 0.0024,1.2 ; 1.0,1.52 ]  InitialFluxes=[ 0.8 , -0.8 , 0.7 ]  BreakLoop=off  DiscreteSolver=Trapezoidal iterative  DataType=off  TransfoNumber=1
  BUS1 : spsThreePhaseVIMeasurementLib/Three-Phase V-I Measurement  VoltageMeasurement=phase-to-ground  SetLabelV=off  LabelV=Vabc  Vpu=off  VpuLL=off  CurrentMeasurement=yes  SetLabelI=off  LabelI=Iabc  Ipu=off  Pbase=100e6  Vbase=500e3  OutputType=Complex  PhasorSimulation=off  PSBequivalent=0
  Mux1 : Mux  Inputs=2
  Scope1 : Scope
  Three-Phase Series RLC Load : spsThreePhaseSeriesRLCLoadLib/Three-Phase Series RLC Load  LConnTagsString=A|B|C  Configuration=Y (grounded)  NominalVoltage=1000  Vabc=[1e3 1e3 1e3]  Vabcp=[1e3 1e3 1e3]  NominalFrequency=60  UnbalancedPower=off  ActivePower=10e3  InductivePower=100  CapacitivePower=100  Pabc=[10e3 9e3 11e3]  QLabc=[100 90 110]  QCabc=[100 90 110]  Pabcp=[10e3 9e3 11e3]  QLabcp=[100 90 110]  QCabcp=[100 90 110]  Measurements=None  LoadType=constant Z
  A : PMIOPort  Side=Left
  B : PMIOPort  Port=2  Side=Left
  C : PMIOPort  Port=3  Side=Left
  wires:
  BUS1/2 -> Mux1/2
  BUS1/1 -> Mux1/1
  Mux1/1 -> Scope1/1
  connections:
  33/11KV Transformer 1/RConn3 -- BUS1/LConn3
  33/11KV Transformer 1/RConn1 -- BUS1/LConn1
  BUS1/RConn2 -- Three-Phase Series RLC Load/LConn2
  BUS1/RConn3 -- Three-Phase Series RLC Load/LConn3
  33/11KV Transformer 1/RConn2 -- BUS1/LConn2
  BUS1/RConn1 -- Three-Phase Series RLC Load/LConn1
  33/11KV Transformer 1/LConn1 -- A/RConn1
  33/11KV Transformer 1/LConn3 -- C/RConn1
  33/11KV Transformer 1/LConn2 -- B/RConn1

== system Campus_Power_System_updated/Law ==
  33/11KV Transformer 1 : spsThreePhaseTransformerTwoWindingsLib/Three-Phase Transformer (Two Windings)  Winding1Connection=Yg  Winding2Connection=Yg  CoreType=Three single-phase transformers  SetSaturation=off  Hysteresis=off  DataFile='hysteresis'  SetInitialFlux=off  Measurements=None  UNITS=pu  NominalPower=[ 250e6 , 50 ]  Winding1=[33e3 , 0.002 , 0.08 ]  Winding2=[ 11e3 , 0.002 , 0.08 ]  Rm=500  Lm=500  L0=0.5  Saturation=[ 0,0 ; 0.0024,1.2 ; 1.0,1.52 ]  InitialFluxes=[ 0.8 , -0.8 , 0.7 ]  BreakLoop=off  DiscreteSolver=Trapezoidal iterative  DataType=off  TransfoNumber=1
  BUS1 : spsThreePhaseVIMeasurementLib/Three-Phase V-I Measurement  VoltageMeasurement=phase-to-ground  SetLabelV=off  LabelV=Vabc  Vpu=off  VpuLL=off  CurrentMeasurement=yes  SetLabelI=off  LabelI=Iabc  Ipu=off  Pbase=100e6  Vbase=500e3  OutputType=Complex  PhasorSimulation=off  PSBequivalent=0
  Mux1 : Mux  Inputs=2
  Scope1 : Scope
  Three-Phase Series RLC Load : spsThreePhaseSeriesRLCLoadLib/Three-Phase Series RLC Load  LConnTagsString=A|B|C  Configuration=Y (grounded)  NominalVoltage=1000  Vabc=[1e3 1e3 1e3]  Vabcp=[1e3 1e3 1e3]  NominalFrequency=60  UnbalancedPower=off  ActivePower=10e3  InductivePower=100  CapacitivePower=100  Pabc=[10e3 9e3 11e3]  QLabc=[100 90 110]  QCabc=[100 90 110]  Pabcp=[10e3 9e3 11e3]  QLabcp=[100 90 110]  QCabcp=[100 90 110]  Measurements=None  LoadType=constant Z
  A : PMIOPort  Side=Left
  B : PMIOPort  Port=2  Side=Left
  C : PMIOPort  Port=3  Side=Left
  wires:
  BUS1/2 -> Mux1/2
  BUS1/1 -> Mux1/1
  Mux1/1 -> Scope1/1
  connections:
  33/11KV Transformer 1/RConn3 -- BUS1/LConn3
  33/11KV Transformer 1/RConn1 -- BUS1/LConn1
  BUS1/RConn2 -- Three-Phase Series RLC Load/LConn2
  BUS1/RConn3 -- Three-Phase Series RLC Load/LConn3
  33/11KV Transformer 1/RConn2 -- BUS1/LConn2
  BUS1/RConn1 -- Three-Phase Series RLC Load/LConn1
  33/11KV Transformer 1/LConn1 -- A/RConn1
  33/11KV Transformer 1/LConn3 -- C/RConn1
  33/11KV Transformer 1/LConn2 -- B/RConn1

== system Campus_Power_System_updated/Library ==
  33/11KV Transformer 1 : spsThreePhaseTransformerTwoWindingsLib/Three-Phase Transformer (Two Windings)  Winding1Connection=Yg  Winding2Connection=Yg  CoreType=Three single-phase transformers  SetSaturation=off  Hysteresis=off  DataFile='hysteresis'  SetInitialFlux=off  Measurements=None  UNITS=pu  NominalPower=[ 250e6 , 50 ]  Winding1=[33e3 , 0.002 , 0.08 ]  Winding2=[ 11e3 , 0.002 , 0.08 ]  Rm=500  Lm=500  L0=0.5  Saturation=[ 0,0 ; 0.0024,1.2 ; 1.0,1.52 ]  InitialFluxes=[ 0.8 , -0.8 , 0.7 ]  BreakLoop=off  DiscreteSolver=Trapezoidal iterative  DataType=off  TransfoNumber=1
  BUS1 : spsThreePhaseVIMeasurementLib/Three-Phase V-I Measurement  VoltageMeasurement=phase-to-ground  SetLabelV=off  LabelV=Vabc  Vpu=off  VpuLL=off  CurrentMeasurement=yes  SetLabelI=off  LabelI=Iabc  Ipu=off  Pbase=100e6  Vbase=500e3  OutputType=Complex  PhasorSimulation=off  PSBequivalent=0
  Mux1 : Mux  Inputs=2
  Scope1 : Scope
  Three-Phase Series RLC Load : spsThreePhaseSeriesRLCLoadLib/Three-Phase Series RLC Load  LConnTagsString=A|B|C  Configuration=Y (grounded)  NominalVoltage=1000  Vabc=[1e3 1e3 1e3]  Vabcp=[1e3 1e3 1e3]  NominalFrequency=60  UnbalancedPower=off  ActivePower=10e3  InductivePower=100  CapacitivePower=100  Pabc=[10e3 9e3 11e3]  QLabc=[100 90 110]  QCabc=[100 90 110]  Pabcp=[10e3 9e3 11e3]  QLabcp=[100 90 110]  QCabcp=[100 90 110]  Measurements=None  LoadType=constant Z
  A : PMIOPort  Side=Left
  B : PMIOPort  Port=2  Side=Left
  C : PMIOPort  Port=3  Side=Left
  wires:
  BUS1/2 -> Mux1/2
  BUS1/1 -> Mux1/1
  Mux1/1 -> Scope1/1
  connections:
  33/11KV Transformer 1/RConn3 -- BUS1/LConn3
  33/11KV Transformer 1/RConn1 -- BUS1/LConn1
  BUS1/RConn2 -- Three-Phase Series RLC Load/LConn2
  BUS1/RConn3 -- Three-Phase Series RLC Load/LConn3
  33/11KV Transformer 1/RConn2 -- BUS1/LConn2
  BUS1/RConn1 -- Three-Phase Series RLC Load/LConn1
  33/11KV Transformer 1/LConn1 -- A/RConn1
  33/11KV Transformer 1/LConn3 -- C/RConn1
  33/11KV Transformer 1/LConn2 -- B/RConn1

== system Campus_Power_System_updated/Main Auditorium ==
  33/11KV Transformer 1 : spsThreePhaseTransformerTwoWindingsLib/Three-Phase Transformer (Two Windings)  Winding1Connection=Yg  Winding2Connection=Yg  CoreType=Three single-phase transformers  SetSaturation=off  Hysteresis=off  DataFile='hysteresis'  SetInitialFlux=off  Measurements=None  UNITS=pu  NominalPower=[ 250e6 , 50 ]  Winding1=[33e3 , 0.002 , 0.08 ]  Winding2=[ 11e3 , 0.002 , 0.08 ]  Rm=500  Lm=500  L0=0.5  Saturation=[ 0,0 ; 0.0024,1.2 ; 1.0,1.52 ]  InitialFluxes=[ 0.8 , -0.8 , 0.7 ]  BreakLoop=off  DiscreteSolver=Trapezoidal iterative  DataType=off  TransfoNumber=1
  BUS1 : spsThreePhaseVIMeasurementLib/Three-Phase V-I Measurement  VoltageMeasurement=phase-to-ground  SetLabelV=off  LabelV=Vabc  Vpu=off  VpuLL=off  CurrentMeasurement=yes  SetLabelI=off  LabelI=Iabc  Ipu=off  Pbase=100e6  Vbase=500e3  OutputType=Complex  PhasorSimulation=off  PSBequivalent=0
  Mux1 : Mux  Inputs=2
  Scope1 : Scope
  Three-Phase Series RLC Load : spsThreePhaseSeriesRLCLoadLib/Three-Phase Series RLC Load  LConnTagsString=A|B|C  Configuration=Y (grounded)  NominalVoltage=1000  Vabc=[1e3 1e3 1e3]  Vabcp=[1e3 1e3 1e3]  NominalFrequency=60  UnbalancedPower=off  ActivePower=10e3  InductivePower=100  CapacitivePower=100  Pabc=[10e3 9e3 11e3]  QLabc=[100 90 110]  QCabc=[100 90 110]  Pabcp=[10e3 9e3 11e3]  QLabcp=[100 90 110]  QCabcp=[100 90 110]  Measurements=None  LoadType=constant Z
  A : PMIOPort  Side=Left
  B : PMIOPort  Port=2  Side=Left
  C : PMIOPort  Port=3  Side=Left
  wires:
  BUS1/2 -> Mux1/2
  BUS1/1 -> Mux1/1
  Mux1/1 -> Scope1/1
  connections:
  33/11KV Transformer 1/RConn3 -- BUS1/LConn3
  33/11KV Transformer 1/RConn1 -- BUS1/LConn1
  BUS1/RConn2 -- Three-Phase Series RLC Load/LConn2
  BUS1/RConn3 -- Three-Phase Series RLC Load/LConn3
  33/11KV Transformer 1/RConn2 -- BUS1/LConn2
  BUS1/RConn1 -- Three-Phase Series RLC Load/LConn1
  33/11KV Transformer 1/LConn1 -- A/RConn1
  33/11KV Transformer 1/LConn3 -- C/RConn1
  33/11KV Transformer 1/LConn2 -- B/RConn1

== system Campus_Power_System_updated/Mareire Hall ==
  33/11KV Transformer 1 : spsThreePhaseTransformerTwoWindingsLib/Three-Phase Transformer (Two Windings)  Winding1Connection=Yg  Winding2Connection=Yg  CoreType=Three single-phase transformers  SetSaturation=off  Hysteresis=off  DataFile='hysteresis'  SetInitialFlux=off  Measurements=None  UNITS=pu  NominalPower=[ 250e6 , 50 ]  Winding1=[33e3 , 0.002 , 0.08 ]  Winding2=[ 11e3 , 0.002 , 0.08 ]  Rm=500  Lm=500  L0=0.5  Saturation=[ 0,0 ; 0.0024,1.2 ; 1.0,1.52 ]  InitialFluxes=[ 0.8 , -0.8 , 0.7 ]  BreakLoop=off  DiscreteSolver=Trapezoidal iterative  DataType=off  TransfoNumber=1
  BUS1 : spsThreePhaseVIMeasurementLib/Three-Phase V-I Measurement  VoltageMeasurement=phase-to-ground  SetLabelV=off  LabelV=Vabc  Vpu=off  VpuLL=off  CurrentMeasurement=yes  SetLabelI=off  LabelI=Iabc  Ipu=off  Pbase=100e6  Vbase=500e3  OutputType=Complex  PhasorSimulation=off  PSBequivalent=0
  Mux1 : Mux  Inputs=2
  Scope1 : Scope
  Three-Phase Series RLC Load : spsThreePhaseSeriesRLCLoadLib/Three-Phase Series RLC Load  LConnTagsString=A|B|C  Configuration=Y (grounded)  NominalVoltage=1000  Vabc=[1e3 1e3 1e3]  Vabcp=[1e3 1e3 1e3]  NominalFrequency=60  UnbalancedPower=off  ActivePower=10e3  InductivePower=100  CapacitivePower=100  Pabc=[10e3 9e3 11e3]  QLabc=[100 90 110]  QCabc=[100 90 110]  Pabcp=[10e3 9e3 11e3]  QLabcp=[100 90 110]  QCabcp=[100 90 110]  Measurements=None  LoadType=constant Z
  A : PMIOPort  Side=Left
  B : PMIOPort  Port=2  Side=Left
  C : PMIOPort  Port=3  Side=Left
  wires:
  BUS1/2 -> Mux1/2
  BUS1/1 -> Mux1/1
  Mux1/1 -> Scope1/1
  connections:
  33/11KV Transformer 1/RConn3 -- BUS1/LConn3
  33/11KV Transformer 1/RConn1 -- BUS1/LConn1
  BUS1/RConn2 -- Three-Phase Series RLC Load/LConn2
  BUS1/RConn3 -- Three-Phase Series RLC Load/LConn3
  33/11KV Transformer 1/RConn2 -- BUS1/LConn2
  BUS1/RConn1 -- Three-Phase Series RLC Load/LConn1
  33/11KV Transformer 1/LConn1 -- A/RConn1
  33/11KV Transformer 1/LConn3 -- C/RConn1
  33/11KV Transformer 1/LConn2 -- B/RConn1

== system Campus_Power_System_updated/Medical Quarters ==
  33/11KV Transformer 1 : spsThreePhaseTransformerTwoWindingsLib/Three-Phase Transformer (Two Windings)  Winding1Connection=Yg  Winding2Connection=Yg  CoreType=Three single-phase transformers  SetSaturation=off  Hysteresis=off  DataFile='hysteresis'  SetInitialFlux=off  Measurements=None  UNITS=pu  NominalPower=[ 250e6 , 50 ]  Winding1=[33e3 , 0.002 , 0.08 ]  Winding2=[ 11e3 , 0.002 , 0.08 ]  Rm=500  Lm=500  L0=0.5  Saturation=[ 0,0 ; 0.0024,1.2 ; 1.0,1.52 ]  InitialFluxes=[ 0.8 , -0.8 , 0.7 ]  BreakLoop=off  DiscreteSolver=Trapezoidal iterative  DataType=off  TransfoNumber=1
  BUS1 : spsThreePhaseVIMeasurementLib/Three-Phase V-I Measurement  VoltageMeasurement=phase-to-ground  SetLabelV=off  LabelV=Vabc  Vpu=off  VpuLL=off  CurrentMeasurement=yes  SetLabelI=off  LabelI=Iabc  Ipu=off  Pbase=100e6  Vbase=500e3  OutputType=Complex  PhasorSimulation=off  PSBequivalent=0
  Mux1 : Mux  Inputs=2
  Scope1 : Scope
  Three-Phase Series RLC Load : spsThreePhaseSeriesRLCLoadLib/Three-Phase Series RLC Load  LConnTagsString=A|B|C  Configuration=Y (grounded)  NominalVoltage=1000  Vabc=[1e3 1e3 1e3]  Vabcp=[1e3 1e3 1e3]  NominalFrequency=60  UnbalancedPower=off  ActivePower=10e3  InductivePower=100  CapacitivePower=100  Pabc=[10e3 9e3 11e3]  QLabc=[100 90 110]  QCabc=[100 90 110]  Pabcp=[10e3 9e3 11e3]  QLabcp=[100 90 110]  QCabcp=[100 90 110]  Measurements=None  LoadType=constant Z
  A : PMIOPort  Side=Left
  B : PMIOPort  Port=2  Side=Left
  C : PMIOPort  Port=3  Side=Left
  wires:
  BUS1/2 -> Mux1/2
  BUS1/1 -> Mux1/1
  Mux1/1 -> Scope1/1
  connections:
  33/11KV Transformer 1/RConn3 -- BUS1/LConn3
  33/11KV Transformer 1/RConn1 -- BUS1/LConn1
  BUS1/RConn2 -- Three-Phase Series RLC Load/LConn2
  BUS1/RConn3 -- Three-Phase Series RLC Load/LConn3
  33/11KV Transformer 1/RConn2 -- BUS1/LConn2
  BUS1/RConn1 -- Three-Phase Series RLC Load/LConn1
  33/11KV Transformer 1/LConn1 -- A/RConn1
  33/11KV Transformer 1/LConn3 -- C/RConn1
  33/11KV Transformer 1/LConn2 -- B/RConn1

== system Campus_Power_System_updated/Moremi Hall ==
  33/11KV Transformer 1 : spsThreePhaseTransformerTwoWindingsLib/Three-Phase Transformer (Two Windings)  Winding1Connection=Yg  Winding2Connection=Yg  CoreType=Three single-phase transformers  SetSaturation=off  Hysteresis=off  DataFile='hysteresis'  SetInitialFlux=off  Measurements=None  UNITS=pu  NominalPower=[ 250e6 , 50 ]  Winding1=[33e3 , 0.002 , 0.08 ]  Winding2=[ 11e3 , 0.002 , 0.08 ]  Rm=500  Lm=500  L0=0.5  Saturation=[ 0,0 ; 0.0024,1.2 ; 1.0,1.52 ]  InitialFluxes=[ 0.8 , -0.8 , 0.7 ]  BreakLoop=off  DiscreteSolver=Trapezoidal iterative  DataType=off  TransfoNumber=1
  BUS1 : spsThreePhaseVIMeasurementLib/Three-Phase V-I Measurement  VoltageMeasurement=phase-to-ground  SetLabelV=off  LabelV=Vabc  Vpu=off  VpuLL=off  CurrentMeasurement=yes  SetLabelI=off  LabelI=Iabc  Ipu=off  Pbase=100e6  Vbase=500e3  OutputType=Complex  PhasorSimulation=off  PSBequivalent=0
  Mux1 : Mux  Inputs=2
  Scope1 : Scope
  Three-Phase Series RLC Load : spsThreePhaseSeriesRLCLoadLib/Three-Phase Series RLC Load  LConnTagsString=A|B|C  Configuration=Y (grounded)  NominalVoltage=1000  Vabc=[1e3 1e3 1e3]  Vabcp=[1e3 1e3 1e3]  NominalFrequency=60  UnbalancedPower=off  ActivePower=10e3  InductivePower=100  CapacitivePower=100  Pabc=[10e3 9e3 11e3]  QLabc=[100 90 110]  QCabc=[100 90 110]  Pabcp=[10e3 9e3 11e3]  QLabcp=[100 90 110]  QCabcp=[100 90 110]  Measurements=None  LoadType=constant Z
  A : PMIOPort  Side=Left
  B : PMIOPort  Port=2  Side=Left
  C : PMIOPort  Port=3  Side=Left
  wires:
  BUS1/2 -> Mux1/2
  BUS1/1 -> Mux1/1
  Mux1/1 -> Scope1/1
  connections:
  33/11KV Transformer 1/RConn3 -- BUS1/LConn3
  33/11KV Transformer 1/RConn1 -- BUS1/LConn1
  BUS1/RConn2 -- Three-Phase Series RLC Load/LConn2
  BUS1/RConn3 -- Three-Phase Series RLC Load/LConn3
  33/11KV Transformer 1/RConn2 -- BUS1/LConn2
  BUS1/RConn1 -- Three-Phase Series RLC Load/LConn1
  33/11KV Transformer 1/LConn1 -- A/RConn1
  33/11KV Transformer 1/LConn3 -- C/RConn1
  33/11KV Transformer 1/LConn2 -- B/RConn1
